simulink model "gm_uz_pmsm_model_6LUT_pd_vnl"  (R2023b)
settings: Solver=FixedStepAuto  StartTime=0.0  StopTime=0.05  RelTol=1e-3
PreLoadFcn:
  | uz_pmsm_model_init_parameter
PostLoadFcn:
  | % Import the data from Excel for a lookup table
  | FluxMapData = readtable('C:\Users\Philipp\ultrazohm\ultrazohm_sw\ip_cores\uz_pmsm_model\FluxMapData_2023-05-26_13-07-57.csv');
  | % Row indices for lookup table
  | d_current_in_d_axis = FluxMapData(8:27,1:end);
  | % Column indices for lookup table
  | q_current_in_d_axis = FluxMapData(29:48,1:end);
  | % Output values for lookup table
  | d_Flux_d_axis = FluxMapData(50:69,1:end);
undefined symbols (not defined in the file or in its folder): ad1, ad2, ad3, ad4, ad5, ad6, aq1, aq2, aq3, aq4, aq5, aq6, d_current_d_Flux, d_current_q_Flux, entkopplung_dynamic, entkopplung_linear, entkopplung_static, Fid1_Giq1, Fid2_Giq2, Flux_d, Flux_q, friction_coefficient, inertia, Ki_Bo_d, Ki_Bo_q, Kp_Bo_d, Kp_Bo_q, L_d, L_q, Ldq, parameter_nachfuerung, polepair, praediktion_entkopplung_nonlinear, psi_pm, q_current_d_Flux, q_current_q_Flux, R_1, simulate_mechanical, simulate_nonlinear_modell, simulate_open_loop, static_friction_torque, tau_sum, ts, ts_regler
libraries: hdlmdlgenlib x21, simulink x2, slpidlib x2
(part 2 of 4)

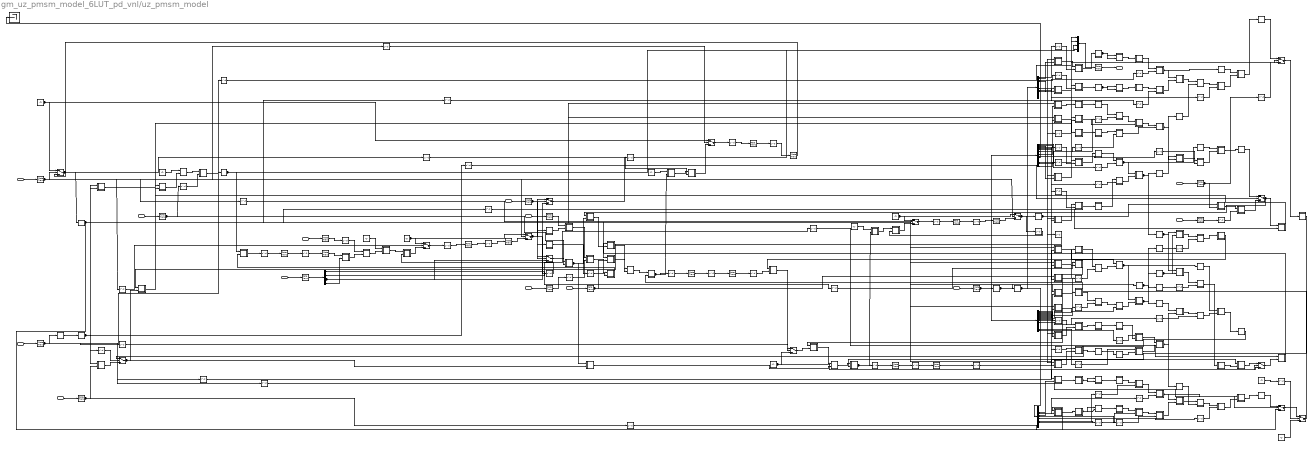
== system gm_uz_pmsm_model_6LUT_pd_vnl/uz_pmsm_model ==
  reset_integrators : Inport  OutDataTypeStr=boolean  PortDimensions=1  SampleTime=2e-06
  simulate_mechanical : Inport  Port=2  OutDataTypeStr=boolean  PortDimensions=1  SampleTime=2e-06
  simulate_nonlinear : Inport  Port=3  OutDataTypeStr=boolean  PortDimensions=1  SampleTime=2e-06
  reciprocal_J : Inport  Port=4  OutDataTypeStr=single  PortDimensions=1  SampleTime=2e-06
  mu : Inport  Port=5  OutDataTypeStr=single  PortDimensions=1  SampleTime=2e-06
  M_n0 : Inport  Port=6  OutDataTypeStr=single  PortDimensions=1  SampleTime=2e-06
  R1 : Inport  Port=7  OutDataTypeStr=single  PortDimensions=1  SampleTime=2e-06
  polepairs : Inport  Port=8  OutDataTypeStr=single  PortDimensions=1  SampleTime=2e-06
  Ld : Inport  Port=9  OutDataTypeStr=single  PortDimensions=1  SampleTime=2e-06
  Lq : Inport  Port=10  OutDataTypeStr=single  PortDimensions=1  SampleTime=2e-06
  psi_pm : Inport  Port=11  OutDataTypeStr=single  PortDimensions=1  SampleTime=2e-06
  fitting_parameters : Inport  Port=12  OutDataTypeStr=single  PortDimensions=[23]  SampleTime=2e-06
  inputs : Inport  Port=13  OutDataTypeStr=single  PortDimensions=[4]  SampleTime=2e-06
  Abs : Subsystem
      mask Display: disp('NFP\nabs');
  Constant : Constant  Value=single(0)  OutDataTypeStr=single  SampleTime=1e-08
  Delay : RateTransition  OutPortSampleTimeOpt=Multiple of input port sample time  OutPortSampleTimeMultiple=200
  Delay1_lowered : RateTransition  OutPortSampleTimeOpt=Multiple of input port sample time  OutPortSampleTimeMultiple=200
  Delay1_lowered1 : RateTransition  OutPortSampleTimeOpt=Multiple of input port sample time  OutPortSampleTimeMultiple=200
  Delay1_lowered2 : RateTransition  OutPortSampleTimeOpt=Multiple of input port sample time  OutPortSampleTimeMultiple=200
  Delay1_lowered_absorbed : Delay  DelayLength=0
  Delay1_lowered_absorbed1 : Delay  DelayLength=0
  Delay1_lowered_absorbed2 : Delay  DelayLength=0
  Delay_absorbed : Delay  DelayLength=0
  Divide : Subsystem
      mask Display: disp('NFP\nmul');
  Divide1 : Subsystem
      mask Display: disp('NFP\nmul');
  Divide_recip : Subsystem
      mask Display: disp('NFP\nmath');
  Factor : Subsystem
      mask Display: disp('NFP\nmul');
  Factor_const : Constant  Value=single(1.5)  OutDataTypeStr=single  SampleTime=1e-08
  From1 : hdlmdlgenlib/Buffer
  From2 : hdlmdlgenlib/Buffer
  From3 : hdlmdlgenlib/Buffer
  Gain : Subsystem
      mask Display: disp('NFP\nmul');
  Gain7 : Subsystem
      mask Display: disp('NFP\nmul');
  Gain71 : Subsystem
      mask Display: disp('NFP\nmul');
  Gain7_const : Constant  Value=single(2e-06)  OutDataTypeStr=single  SampleTime=1e-08
  Gain7_const1 : Constant  Value=single(2e-06)  OutDataTypeStr=single  SampleTime=1e-08
  Gain_const : Constant  Value=single(2e-06)  OutDataTypeStr=single  SampleTime=1e-08
  Gain_unaryminus : Subsystem
      mask Display: disp('NFP\numinus');
  Gain_unaryminus1 : Subsystem
      mask Display: disp('NFP\numinus');
  Goto1 : hdlmdlgenlib/Buffer
  Goto2 : hdlmdlgenlib/Buffer
  Initial_Val : Constant  Value=single(0)  OutDataTypeStr=single  SampleTime=1e-08
  Initial_Val1 : Constant  Value=single(0)  OutDataTypeStr=single  SampleTime=1e-08
  Initial_Val2 : Constant  Value=single(0)  OutDataTypeStr=single  SampleTime=1e-08
  Ldd : hdlmdlgenlib/Buffer
  Log : Subsystem
      mask Display: disp('NFP\nmath');
  Log1 : Subsystem
      mask Display: disp('NFP\nmath');
  Log11 : Subsystem
      mask Display: disp('NFP\nmath');
  Log2 : Subsystem
      mask Display: disp('NFP\nmath');
  Lqq : hdlmdlgenlib/Buffer
  Product : Subsystem
      mask Display: disp('NFP\nmul');
  Product1 : Subsystem
      mask Display: disp('NFP\nmul');
  Product10 : Subsystem
      mask Display: disp('NFP\nmul');
  Product101 : Subsystem
      mask Display: disp('NFP\nmul');
  Product102 : Subsystem
      mask Display: disp('NFP\nmul');
  Product103 : Subsystem
      mask Display: disp('NFP\nmul');
  Product104 : Subsystem
      mask Display: disp('NFP\nmul');
  Product11 : Subsystem
      mask Display: disp('NFP\nmul');
  Product110 : Subsystem
      mask Display: disp('NFP\nmul');
  Product111 : Subsystem
      mask Display: disp('NFP\nmul');
  Product12 : Subsystem
      mask Display: disp('NFP\nmul');
  Product121 : Subsystem
      mask Display: disp('NFP\nmul');
  Product122 : Subsystem
      mask Display: disp('NFP\nmul');
  Product13 : Subsystem
      mask Display: disp('NFP\nmul');
  Product131 : Subsystem
      mask Display: disp('NFP\nmul');
  Product14 : Subsystem
      mask Display: disp('NFP\nmul');
  Product141 : Subsystem
      mask Display: disp('NFP\nmul');
  Product142 : Subsystem
      mask Display: disp('NFP\nmul');
  Product15 : Subsystem
      mask Display: disp('NFP\nmul');
  Product151 : Subsystem
      mask Display: disp('NFP\nmul');
  Product16 : Subsystem
      mask Display: disp('NFP\nmul');
  Product17 : Subsystem
      mask Display: disp('NFP\nmul');
  Product18 : Subsystem
      mask Display: disp('NFP\nmul');
  Product19 : Subsystem
      mask Display: disp('NFP\nmul');
  Product2 : Subsystem
      mask Display: disp('NFP\nmul');
  Product20 : Subsystem
      mask Display: disp('NFP\nmul');
  Product201 : Subsystem
      mask Display: disp('NFP\nmul');
  Product202 : Subsystem
      mask Display: disp('NFP\nmul');
  Product203 : Subsystem
      mask Display: disp('NFP\nmul');
  Product204 : Subsystem
      mask Display: disp('NFP\nmul');
  Product205 : Subsystem
      mask Display: disp('NFP\nmul');
  Product206 : Subsystem
      mask Display: disp('NFP\nmul');
  Product207 : Subsystem
      mask Display: disp('NFP\nmul');
  Product21 : Subsystem
      mask Display: disp('NFP\nmul');
  Product22 : Subsystem
      mask Display: disp('NFP\nmul');
  Product23 : Subsystem
      mask Display: disp('NFP\nmul');
  Product24 : Subsystem
      mask Display: disp('NFP\nmul');
  Product25 : Subsystem
      mask Display: disp('NFP\nmul');
  Product3 : Subsystem
      mask Display: disp('NFP\nmul');
  Product31 : Subsystem
      mask Display: disp('NFP\nmul');
  Product32 : Subsystem
      mask Display: disp('NFP\nmul');
  Product33 : Subsystem
      mask Display: disp('NFP\nmul');
  Product34 : Subsystem
      mask Display: disp('NFP\nmul');
  Product35 : Subsystem
      mask Display: disp('NFP\nmul');
  Product4 : Subsystem
      mask Display: disp('NFP\nmul');
  Product41 : Subsystem
      mask Display: disp('NFP\nmul');
  Product42 : Subsystem
      mask Display: disp('NFP\nmul');
  Product43 : Subsystem
      mask Display: disp('NFP\nmul');
  Product5 : Subsystem
      mask Display: disp('NFP\nmul');
  Product51 : Subsystem
      mask Display: disp('NFP\nmul');
  Product52 : Subsystem
      mask Display: disp('NFP\nmul');
  Product6 : Subsystem
      mask Display: disp('NFP\nmul');
  Product61 : Subsystem
      mask Display: disp('NFP\nmul');
  Product7 : Subsystem
      mask Display: disp('NFP\nmul');
  Product71 : Subsystem
      mask Display: disp('NFP\nmul');
  Product8 : Subsystem
      mask Display: disp('NFP\nmul');
  Product9 : Subsystem
      mask Display: disp('NFP\nmul');
  Product91 : Subsystem
      mask Display: disp('NFP\nmul');
  Product92 : Subsystem
      mask Display: disp('NFP\nmul');
  Reciprocal1_recip : Subsystem
      mask Display: disp('NFP\nmath');
  Reciprocal1_recip1 : Subsystem
      mask Display: disp('NFP\nmath');
  Reciprocal_recip : Subsystem
      mask Display: disp('NFP\nmath');
  Reciprocal_recip1 : Subsystem
      mask Display: disp('NFP\nmath');
  Selector : Selector  IndexOptions=Index vector (dialog)  Indices=double(13)  OutputSizes=double(1)
  Selector1 : Selector  IndexOptions=Index vector (dialog)  Indices=double(14)  OutputSizes=double(1)
  Sign1 : Subsystem
      mask Display: disp('NFP\nsignum');
  Sum : Subsystem
      mask Display: disp('NFP\nadd');
  Sum1 : Subsystem
      mask Display: disp('NFP\nadd');
  Sum10 : Subsystem
      mask Display: disp('NFP\nadd');
  Sum101 : Subsystem
      mask Display: disp('NFP\nadd');
  Sum11 : Subsystem
      mask Display: disp('NFP\nadd');
  Sum12 : Subsystem
      mask Display: disp('NFP\nadd');
  Sum13 : Subsystem
      mask Display: disp('NFP\nadd');
  Sum14 : Subsystem
      mask Display: disp('NFP\nadd');
  Sum2 : Subsystem
      mask Display: disp('NFP\nadd');
  Sum21 : Subsystem
      mask Display: disp('NFP\nadd');
  Sum22 : Subsystem
      mask Display: disp('NFP\nadd');
  Sum23 : Subsystem
      mask Display: disp('NFP\nadd');
  Sum3 : Subsystem
      mask Display: disp('NFP\nadd');
  Sum31 : Subsystem
      mask Display: disp('NFP\nadd');
  Sum32 : Subsystem
      mask Display: disp('NFP\nadd');
  Sum33 : Subsystem
      mask Display: disp('NFP\nadd');
  Sum3_stage2 : Subsystem
      mask Display: disp('NFP\nadd');
  Sum3_stage21 : Subsystem
      mask Display: disp('NFP\nadd');
  Sum3_stage3 : Subsystem
      mask Display: disp('NFP\nadd');
  Sum3_stage31 : Subsystem
      mask Display: disp('NFP\nadd');
  Sum3_stage4 : Subsystem
      mask Display: disp('NFP\nadd');
  Sum4 : Subsystem
      mask Display: disp('NFP\nadd');
  Sum41 : Subsystem
      mask Display: disp('NFP\nadd');
  Sum42 : Subsystem
      mask Display: disp('NFP\nadd');
  Sum4_stage2 : Subsystem
      mask Display: disp('NFP\nadd');
  Sum4_stage3 : Subsystem
      mask Display: disp('NFP\nadd');
  Sum4_stage4 : Subsystem
      mask Display: disp('NFP\nadd');
  Sum5 : Subsystem
      mask Display: disp('NFP\nadd');
  Sum51 : Subsystem
      mask Display: disp('NFP\nadd');
  Sum52 : Subsystem
      mask Display: disp('NFP\nadd');
  Sum53 : Subsystem
      mask Display: disp('NFP\nadd');
  Sum6 : Subsystem
      mask Display: disp('NFP\nadd');
  Sum7 : Subsystem
      mask Display: disp('NFP\nadd');
  Sum71 : Subsystem
      mask Display: disp('NFP\nadd');
  Sum8 : Subsystem
      mask Display: disp('NFP\nadd');
  Switch{,1..6,11} (8 alike) : Switch  Criteria=u2 ~= 0  Threshold=double(0)  OutDataTypeStr=single  SampleTime=1e-08  SaturateOnIntegerOverflow=off  InputSameDT=off
  Tanh : Subsystem
      mask Display: disp('NFP\ntrig');
  Tanh1 : Subsystem
      mask Display: disp('NFP\ntrig');
  Tanh11 : Subsystem
      mask Display: disp('NFP\ntrig');
  Tanh12 : Subsystem
      mask Display: disp('NFP\ntrig');
  Tanh13 : Subsystem
      mask Display: disp('NFP\ntrig');
  Tanh2 : Subsystem
      mask Display: disp('NFP\ntrig');
  Tanh21 : Subsystem
      mask Display: disp('NFP\ntrig');
  Tanh3 : Subsystem
      mask Display: disp('NFP\ntrig');
  Tanh31 : Subsystem
      mask Display: disp('NFP\ntrig');
  Tanh4 : Subsystem
      mask Display: disp('NFP\ntrig');
  Tanh41 : Subsystem
      mask Display: disp('NFP\ntrig');
  Tanh5 : Subsystem
      mask Display: disp('NFP\ntrig');
  Unit Delay : RateTransition  OutPortSampleTimeOpt=Multiple of input port sample time  OutPortSampleTimeMultiple=200
  Unit Delay1 : RateTransition  OutPortSampleTimeOpt=Multiple of input port sample time  OutPortSampleTimeMultiple=200
  Unit Delay1_absorbed : Delay  DelayLength=0
  Unit Delay_absorbed : Delay  DelayLength=0
  crp_out_delay{,1..5} (6 alike) : Delay  DelayLength=double(1)  InitialCondition=0  SampleTime=1e-08
  default_value : Constant  Value=double(1)  OutDataTypeStr=single  SampleTime=1e-08
  delayMatch{,1..49,51..55} (55 alike) : Delay  DelayLength=double(1)  InitialCondition=0  SampleTime=1e-08
  delayMatch50 : Delay  DelayLength=double(97)  InitialCondition=0  SampleTime=1e-08
  fitting_parameters_13_term13 : Terminator
  i_q : hdlmdlgenlib/Buffer
  in0_repeat : RateTransition  Integrity=off  Deterministic=off  OutPortSampleTimeOpt=Multiple of input port sample time  OutPortSampleTimeMultiple=1/200
  in10_repeat : RateTransition  Integrity=off  Deterministic=off  OutPortSampleTimeOpt=Multiple of input port sample time  OutPortSampleTimeMultiple=1/200
  in11_repeat : RateTransition  Integrity=off  Deterministic=off  OutPortSampleTimeOpt=Multiple of input port sample time  OutPortSampleTimeMultiple=1/200
  in12_repeat : RateTransition  Integrity=off  Deterministic=off  OutPortSampleTimeOpt=Multiple of input port sample time  OutPortSampleTimeMultiple=1/200
  in13_repeat : RateTransition  Integrity=off  Deterministic=off  OutPortSampleTimeOpt=Multiple of input port sample time  OutPortSampleTimeMultiple=1/200
  in14_repeat : RateTransition  Integrity=off  Deterministic=off  OutPortSampleTimeOpt=Multiple of input port sample time  OutPortSampleTimeMultiple=1/200
  in15_repeat : RateTransition  Integrity=off  Deterministic=off  OutPortSampleTimeOpt=Multiple of input port sample time  OutPortSampleTimeMultiple=1/200
  in16_repeat : RateTransition  Integrity=off  Deterministic=off  OutPortSampleTimeOpt=Multiple of input port sample time  OutPortSampleTimeMultiple=1/200
  in17_repeat : RateTransition  Integrity=off  Deterministic=off  OutPortSampleTimeOpt=Multiple of input port sample time  OutPortSampleTimeMultiple=1/200
  in18_repeat : RateTransition  Integrity=off  Deterministic=off  OutPortSampleTimeOpt=Multiple of input port sample time  OutPortSampleTimeMultiple=1/200
  in1_repeat : RateTransition  Integrity=off  Deterministic=off  OutPortSampleTimeOpt=Multiple of input port sample time  OutPortSampleTimeMultiple=1/200
  in2_repeat : RateTransition  Integrity=off  Deterministic=off  OutPortSampleTimeOpt=Multiple of input port sample time  OutPortSampleTimeMultiple=1/200
  in3_repeat : RateTransition  Integrity=off  Deterministic=off  OutPortSampleTimeOpt=Multiple of input port sample time  OutPortSampleTimeMultiple=1/200
  in4_repeat : RateTransition  Integrity=off  Deterministic=off  OutPortSampleTimeOpt=Multiple of input port sample time  OutPortSampleTimeMultiple=1/200
  in5_repeat : RateTransition  Integrity=off  Deterministic=off  OutPortSampleTimeOpt=Multiple of input port sample time  OutPortSampleTimeMultiple=1/200
  in6_repeat : RateTransition  Integrity=off  Deterministic=off  OutPortSampleTimeOpt=Multiple of input port sample time  OutPortSampleTimeMultiple=1/200
  in7_repeat : RateTransition  Integrity=off  Deterministic=off  OutPortSampleTimeOpt=Multiple of input port sample time  OutPortSampleTimeMultiple=1/200
  in8_repeat : RateTransition  Integrity=off  Deterministic=off  OutPortSampleTimeOpt=Multiple of input port sample time  OutPortSampleTimeMultiple=1/200
  in9_repeat : RateTransition  Integrity=off  Deterministic=off  OutPortSampleTimeOpt=Multiple of input port sample time  OutPortSampleTimeMultiple=1/200
  mux : Mux
  psi_d_approx : hdlmdlgenlib/Buffer
  psi_q_approx : hdlmdlgenlib/Buffer
  reset_in : Switch  Criteria=u2 ~= 0  Threshold=double(0)  OutDataTypeStr=single  SampleTime=1e-08  SaturateOnIntegerOverflow=off  InputSameDT=off
  reset_in1 : Switch  Criteria=u2 ~= 0  Threshold=double(0)  OutDataTypeStr=single  SampleTime=1e-08  SaturateOnIntegerOverflow=off  InputSameDT=off
  reset_in2 : Switch  Criteria=u2 ~= 0  Threshold=double(0)  OutDataTypeStr=single  SampleTime=1e-08  SaturateOnIntegerOverflow=off  InputSameDT=off
  reset_out : Switch  Criteria=u2 ~= 0  Threshold=double(0)  OutDataTypeStr=single  SampleTime=1e-08  SaturateOnIntegerOverflow=off  InputSameDT=off
  reset_out1 : Switch  Criteria=u2 ~= 0  Threshold=double(0)  OutDataTypeStr=single  SampleTime=1e-08  SaturateOnIntegerOverflow=off  InputSameDT=off
  reset_out2 : Switch  Criteria=u2 ~= 0  Threshold=double(0)  OutDataTypeStr=single  SampleTime=1e-08  SaturateOnIntegerOverflow=off  InputSameDT=off
  select_signal : Constant  Value=double(1)  OutDataTypeStr=boolean  SampleTime=1e-08
  t : RateTransition  OutPortSampleTimeOpt=Multiple of input port sample time  OutPortSampleTimeMultiple=200
  t{1..4} (4 alike) : Demux  Outputs=23
  t{6..16} (11 alike) : hdlmdlgenlib/Buffer
  t5 : Demux
  zero_protection : Switch  Criteria=u2 ~= 0  Threshold=double(0)  OutDataTypeStr=single  SampleTime=1e-08  SaturateOnIntegerOverflow=off  InputSameDT=off
  outputs : Outport  SampleTime=2e-06
  wires:
  default_value/1 -> zero_protection/3
  zero_protection/1 -> Divide1/2(In2)
  reset_out1/1 -> Switch/1, Switch11/1, Sign1/1(In1), Abs/1(In1), delayMatch54/1
  delayMatch55/1 -> reset_in1/2
  reset_out/1 -> delayMatch51/1, t9/1
  select_signal/1 -> delayMatch50/1
  Switch1/1 -> zero_protection/1
  delayMatch48/1 -> Switch1/2
  Selector1/1 -> delayMatch39/1
  Switch11/1 -> delayMatch36/1
  delayMatch34/1 -> mux/1
  delayMatch35/1 -> mux/2
  From3/1 -> delayMatch14/1, delayMatch30/1
  delayMatch52/1 -> reset_in/2
  reset_out2/1 -> delayMatch26/1, t11/1
  delayMatch41/1 -> Switch4/2
  delayMatch24/1 -> Switch2/2
  delayMatch30/1 -> Switch5/2
  Selector/1 -> delayMatch7/1
  delayMatch50/1 -> zero_protection/2
  Gain/1(Out1) -> Sum32/1(In1)
  Sum3_stage4/1(Out1) -> Divide/1(In1)
  Sum3_stage31/1(Out1) -> Sum3_stage4/1(In1)
  Sum3_stage21/1(Out1) -> Sum3_stage31/1(In1)
  Divide_recip/1(Out1) -> Divide/2(In2)
  Sum53/1(Out1) -> reset_in2/3
  Product43/1(Out1) -> Sum3_stage21/2(In2)
  Product35/1(Out1) -> Sum33/1(In1)
  Sum33/1(Out1) -> Factor/2(In2)
  Sum8/1(Out1) -> crp_out_delay2/1
  Product42/1(Out1) -> Sum8/2(In2)
  Sum52/1(Out1) -> Product42/1(In1)
  Product122/1(Out1) -> Sum52/1(In1)
  Abs/1(Out1) -> Product122/2(In2)
  Sum32/1(Out1) -> reset_in1/3
  Product111/1(Out1) -> Gain/2(In2)
  Sum14/1(Out1) -> Product111/2(In2)
  Sign1/1(Out1) -> delayMatch38/1
  Product131/1(Out1) -> Product34/1(In1), Product22/2(In2)
  Sum42/1(Out1) -> Sum23/1(In1), t16/1
  Sum23/1(Out1) -> t10/1, t15/1
  Product206/1(Out1) -> Product207/1(In1)
  Product121/1(Out1) -> Switch3/1
  Sum4_stage4/1(Out1) -> Divide1/1(In1)
  Sum4_stage3/1(Out1) -> Sum4_stage4/1(In1)
  Sum4_stage2/1(Out1) -> Sum4_stage3/1(In1)
  Sum51/1(Out1) -> reset_in/3
  Product25/1(Out1) -> Tanh13/1(In1)
  Tanh13/1(Out1) -> Product151/1(In1), Product151/2(In2)
  Product151/1(Out1) -> Reciprocal1_recip1/1(In1)
  Reciprocal1_recip1/1(Out1) -> Product33/1(In1)
  Sum41/1(Out1) -> Sum22/2(In2)
  Sum22/1(Out1) -> Product204/1(In1)
  Product204/1(Out1) -> Product205/1(In1)
  Product202/1(Out1) -> Product203/1(In1)
  Tanh12/1(Out1) -> Product32/1(In1)
  Product24/1(Out1) -> Tanh12/1(In1)
  Sum13/1(Out1) -> Sum23/2(In2)
  Product61/1(Out1) -> Sum13/2(In2)
  Product52/1(Out1) -> Sum42/1(In1)
  Product110/1(Out1) -> Sum42/2(In2)
  Tanh5/1(Out1) -> Product110/1(In1)
  Product19/1(Out1) -> Tanh5/1(In1)
  Tanh21/1(Out1) -> Log11/1(In1)
  Log11/1(Out1) -> Product91/2(In2)
  Product91/1(Out1) -> Sum5/2(In2)
  Tanh41/1(Out1) -> Log2/1(In1)
  Log2/1(Out1) -> Product41/2(In2)
  Product41/1(Out1) -> Sum5/1(In1)
  Sum12/1(Out1) -> Sum10/1(In1), Sum22/1(In1)
  Reciprocal_recip1/1(Out1) -> Product18/1(In1)
  Product142/1(Out1) -> Reciprocal_recip1/1(In1)
  Tanh31/1(Out1) -> Product142/1(In1), Product142/2(In2)
  Product17/1(Out1) -> Tanh31/1(In1)
  Product16/1(Out1) -> Tanh4/1(In1)
  Sum4/1(Out1) -> Product16/1(In1)
  Tanh4/1(Out1) -> Product141/1(In1), Product141/2(In2)
  Product141/1(Out1) -> Reciprocal_recip/1(In1)
  Reciprocal_recip/1(Out1) -> Product14/1(In1)
  Product14/1(Out1) -> Sum2/1(In1), t12/1
  Product102/1(Out1) -> Product103/1(In1)
  Sum3_stage2/1(Out1) -> Sum3_stage3/1(In1)
  Product10/1(Out1) -> Product101/1(In1)
  Product13/1(Out1) -> Sum21/1(In1), t14/1
  Sum21/1(Out1) -> t8/1, t13/1
  Tanh11/1(Out1) -> Product31/1(In1)
  Product23/1(Out1) -> Tanh11/1(In1)
  Sum11/1(Out1) -> Product23/1(In1)
  Product7/1(Out1) -> Sum3_stage2/2(In2)
  Product8/1(Out1) -> Product7/1(In1)
  Product51/1(Out1) -> Tanh3/1(In1)
  Tanh3/1(Out1) -> Log1/1(In1)
  Log1/1(Out1) -> Product12/1(In1)
  Product12/1(Out1) -> Sum3_stage3/2(In2)
  Product4/1(Out1) -> Tanh2/1(In1)
  Tanh2/1(Out1) -> Log/1(In1)
  Log/1(Out1) -> Product6/1(In1)
  Product6/1(Out1) -> Sum3_stage2/1(In1)
  Product/1(Out1) -> Tanh/1(In1)
  Sum3/1(Out1) -> Product/1(In1)
  Tanh/1(Out1) -> Product13/1(In1)
  Product201/1(Out1) -> Gain_unaryminus/1(In1)
  Product20/1(Out1) -> Product201/1(In1)
  Product11/1(Out1) -> Switch4/1
  Sum/1(Out1) -> Switch5/3
  Product5/1(Out1) -> Sum/1(In1)
  Reciprocal1_recip/1(Out1) -> Product3/1(In1)
  Product15/1(Out1) -> Reciprocal1_recip/1(In1)
  Tanh1/1(Out1) -> Product15/1(In1), Product15/2(In2)
  Product21/1(Out1) -> Tanh1/1(In1)
  Sum1/1(Out1) -> Product21/1(In1)
  Product9/1(Out1) -> Sum4_stage4/2(In2)
  Product1/1(Out1) -> Switch6/3
  Product2/1(Out1) -> Sum33/2(In2)
  Gain7_const1/1 -> Gain71/1(In1)
  Factor_const/1 -> Factor/1(In1)
  Gain_const/1 -> Gain/1(In1)
  Gain7_const/1 -> Gain7/1(In1)
  t5/2 -> delayMatch42/1
  t5/1 -> delayMatch/1
  t4/22 -> delayMatch10/1
  t4/21 -> delayMatch12/1
  t4/14 -> delayMatch13/1
  t4/10 -> delayMatch6/1
  t4/7 -> delayMatch5/1
  t4/5 -> delayMatch11/1
  t4/2 -> delayMatch9/1
  t3/18 -> delayMatch43/1
  t3/17 -> delayMatch45/1
  t3/14 -> delayMatch47/1
  t3/12 -> delayMatch46/1
  t3/9 -> delayMatch44/1
  t2/16 -> delayMatch16/1
  t2/15 -> delayMatch18/1
  t2/13 -> delayMatch22/1
  t2/5 -> delayMatch17/1
  t2/2 -> delayMatch15/1
  t1/23 -> delayMatch20/1
  t1/20 -> delayMatch19/1
  t1/19 -> delayMatch21/1
  t1/14 -> fitting_parameters_13_term13/1
  t1/13 -> delayMatch28/1
  t1/5 -> delayMatch3/1
  t1/4 -> delayMatch4/1
  t1/2 -> delayMatch1/1
  t1/1 -> delayMatch2/1
  delayMatch37/1 -> Sum52/2(In2)
  delayMatch53/1 -> Product111/1(In1)
  delayMatch33/1 -> Product92/2(In2)
  delayMatch8/1 -> Product121/2(In2)
  delayMatch27/1 -> reset_in2/2
  delayMatch40/1 -> Product11/1(In1)
  delayMatch29/1 -> Sum/2(In2)
  delayMatch25/1 -> Switch2/3
  delayMatch49/1 -> Switch1/3
  delayMatch23/1 -> Switch3/2
  t5/4 -> Sum14/2(In2)
  t5/3 -> Switch/3, Switch11/3
  delayMatch42/1 -> Sum4_stage2/1(In1)
  delayMatch/1 -> Sum3_stage21/1(In1)
  Divide/1(Out1) -> crp_out_delay/1, Gain71/2(In2)
  Gain71/1(Out1) -> Sum53/1(In1)
  reset_in2/1 -> crp_out_delay1/1
  Initial_Val2/1 -> reset_in2/1, reset_out2/1
  delayMatch26/1 -> Sum53/2(In2)
  t11/1 -> delayMatch32/1, delayMatch34/1, Sum1/1(In1), Product5/1(In1), Sum3/1(In1), Sum11/1(In1), Sum4/1(In1), Sum31/1(In1), Sum6/1(In1), Product43/2(In2)
  delayMatch32/1 -> Product2/1(In1)
  delayMatch31/1 -> Product35/2(In2)
  Factor/1(Out1) -> Product92/1(In1)
  Product92/1(Out1) -> i_q/1
  i_q/1 -> mux/3, Sum8/1(In1)
  delayMatch54/1 -> Sum32/2(In2)
  reset_in1/1 -> crp_out_delay5/1
  Initial_Val1/1 -> reset_in1/1, reset_out1/1
  delayMatch38/1 -> Product42/2(In2)
  delayMatch36/1 -> mux/4
  Switch/1 -> Product131/1(In1)
  Product34/1(Out1) -> Sum3_stage4/2(In2)
  Switch6/1 -> Product2/2(In2), Product34/2(In2)
  psi_q_approx/1 -> Switch6/1
  Sum101/1(Out1) -> psi_q_approx/1
  t16/1 -> Sum101/1(In1)
  t15/1 -> Product202/1(In1)
  t10/1 -> Product20/2(In2), Product206/2(In2)
  Product207/1(Out1) -> Gain_unaryminus1/1(In1)
  Gain_unaryminus1/1(Out1) -> Product121/1(In1)
  Switch3/1 -> Sum3_stage31/2(In2)
  Constant/1 -> Switch4/3, Switch3/3
  Switch4/1 -> Sum4_stage2/2(In2)
  Divide1/1(Out1) -> crp_out_delay3/1, Gain7/2(In2)
  Gain7/1(Out1) -> Sum51/1(In1)
  reset_in/1 -> crp_out_delay4/1
  Initial_Val/1 -> reset_in/1, reset_out/1
  delayMatch51/1 -> Sum51/2(In2)
  t9/1 -> delayMatch31/1, delayMatch35/1, Product1/1(In1), Product9/1(In1), Product4/1(In1), Product51/1(In1), Product8/1(In1), Product8/2(In2), Product17/1(In1), Product19/1(In1), Product52/1(In1), Product61/1(In1), Product24/1(In1), Product25/1(In1)
  Product33/1(Out1) -> Sum41/1(In1)
  Product205/1(Out1) -> Sum10/2(In2)
  t6/1 -> Product204/2(In2)
  Sum5/1(Out1) -> Product202/2(In2), t6/1
  Product203/1(Out1) -> Sum101/2(In2)
  delayMatch10/1 -> Product41/1(In1)
  delayMatch12/1 -> Product91/1(In1)
  delayMatch13/1 -> Product203/2(In2)
  t4/12 -> Product61/2(In2)
  t4/11 -> Product24/2(In2)
  delayMatch6/1 -> Product32/2(In2)
  t4/9 -> Product52/2(In2)
  t4/8 -> Product19/2(In2)
  delayMatch5/1 -> Product110/2(In2)
  t4/6 -> Sum6/2(In2)
  delayMatch11/1 -> Product104/1(In1)
  t4/3 -> Sum31/2(In2)
  delayMatch9/1 -> Product71/1(In1)
  Product32/1(Out1) -> Sum13/1(In1)
  Product104/1(Out1) -> Tanh21/1(In1)
  Sum6/1(Out1) -> Product104/2(In2)
  Product71/1(Out1) -> Tanh41/1(In1)
  Sum31/1(Out1) -> Product71/2(In2)
  Sum10/1(Out1) -> Lqq/1
  Product18/1(Out1) -> Sum12/1(In1)
  delayMatch43/1 -> Product18/2(In2)
  delayMatch45/1 -> Product33/2(In2)
  delayMatch47/1 -> Product205/2(In2)
  delayMatch46/1 -> Sum41/2(In2)
  t3/11 -> Product25/2(In2)
  delayMatch44/1 -> Sum12/2(In2)
  t3/8 -> Product17/2(In2)
  From1/1 -> t2/1, t3/1
  delayMatch16/1 -> Product14/2(In2)
  delayMatch18/1 -> Product3/2(In2)
  delayMatch22/1 -> Product103/2(In2)
  t2/6 -> Sum1/2(In2)
  delayMatch17/1 -> Product21/2(In2)
  t2/3 -> Sum4/2(In2)
  delayMatch15/1 -> Product16/2(In2)
  t12/1 -> Sum71/1(In1)
  Sum71/1(Out1) -> Ldd/1
  Product103/1(Out1) -> Sum71/2(In2)
  t7/1 -> Product102/2(In2)
  Sum3_stage3/1(Out1) -> Product10/2(In2), t7/1
  Product101/1(Out1) -> Sum7/2(In2)
  Sum7/1(Out1) -> psi_d_approx/1
  t14/1 -> Sum7/1(In1)
  t13/1 -> Product10/1(In1)
  Product31/1(Out1) -> Sum21/2(In2)
  delayMatch20/1 -> Product7/2(In2)
  delayMatch19/1 -> Product6/2(In2)
  delayMatch21/1 -> Product12/2(In2)
  delayMatch28/1 -> Product101/2(In2)
  t1/11 -> Product51/2(In2)
  t1/8 -> Product4/2(In2)
  t1/6 -> Sum11/2(In2)
  delayMatch3/1 -> Product23/2(In2)
  delayMatch4/1 -> Product31/2(In2)
  t1/3 -> Sum3/2(In2)
  delayMatch1/1 -> Product/2(In2)
  delayMatch2/1 -> Product13/2(In2)
  t8/1 -> Product20/1(In1), Product206/1(In1)
  delayMatch39/1 -> Product201/2(In2)
  From2/1 -> Selector/1, Selector1/1
  Goto1/1 -> From1/1, From2/1
  delayMatch7/1 -> Product207/2(In2)
  Gain_unaryminus/1(Out1) -> Product11/2(In2)
  psi_d_approx/1 -> Switch5/1
  Switch5/1 -> Product35/1(In1), Product22/1(In1)
  delayMatch14/1 -> Switch6/2
  Goto2/1 -> From3/1
  Product22/1(Out1) -> Sum4_stage3/2(In2)
  Sum2/1(Out1) -> Product102/1(In1)
  Product3/1(Out1) -> Sum2/2(In2)
  Ldd/1 -> Switch2/1
  Switch2/1 -> Divide_recip/1(In1)
  Lqq/1 -> Switch1/1
  crp_out_delay5/1 -> Delay1_lowered1/1
  crp_out_delay4/1 -> Delay1_lowered2/1
  crp_out_delay3/1 -> Unit Delay1/1
  crp_out_delay2/1 -> Delay/1
  crp_out_delay1/1 -> Delay1_lowered/1
  crp_out_delay/1 -> Unit Delay/1
  in6_repeat/1 -> delayMatch40/1
  Unit Delay_absorbed/1 -> in6_repeat/1
  Unit Delay/1 -> Unit Delay_absorbed/1
  in9_repeat/1 -> reset_out/3
  Delay1_lowered_absorbed2/1 -> in9_repeat/1
  Delay1_lowered2/1 -> Delay1_lowered_absorbed2/1
  in10_repeat/1 -> delayMatch8/1
  Unit Delay1_absorbed/1 -> in10_repeat/1
  Unit Delay1/1 -> Unit Delay1_absorbed/1
  in14_repeat/1 -> Sum14/1(In1)
  Delay_absorbed/1 -> in14_repeat/1
  Delay/1 -> Delay_absorbed/1
  in15_repeat/1 -> reset_out1/3
  Delay1_lowered_absorbed1/1 -> in15_repeat/1
  Delay1_lowered1/1 -> Delay1_lowered_absorbed1/1
  in17_repeat/1 -> reset_out2/3
  Delay1_lowered_absorbed/1 -> in17_repeat/1
  Delay1_lowered/1 -> Delay1_lowered_absorbed/1
  mux/1 -> t/1
  in18_repeat/1 -> t5/1
  in16_repeat/1 -> delayMatch37/1
  in13_repeat/1 -> delayMatch53/1
  in12_repeat/1 -> Switch/2, Switch11/2
  in11_repeat/1 -> Product131/2(In2), delayMatch33/1
  in8_repeat/1 -> reset_out/2, reset_out2/2, reset_out1/2, delayMatch27/1, delayMatch52/1, delayMatch55/1
  in7_repeat/1 -> Goto1/1, t1/1, t4/1
  in5_repeat/1 -> delayMatch29/1
  in4_repeat/1 -> Product5/2(In2), delayMatch25/1
  in3_repeat/1 -> Product9/2(In2), Product43/1(In1)
  in2_repeat/1 -> Product1/2(In2), delayMatch49/1
  in1_repeat/1 -> Goto2/1, delayMatch23/1, delayMatch24/1, delayMatch41/1, delayMatch48/1
  in0_repeat/1 -> Product122/1(In1)
  t/1 -> outputs/1
  inputs/1 -> in18_repeat/1
  fitting_parameters/1 -> in7_repeat/1
  psi_pm/1 -> in5_repeat/1
  Lq/1 -> in2_repeat/1
  Ld/1 -> in4_repeat/1
  polepairs/1 -> in11_repeat/1
  R1/1 -> in3_repeat/1
  M_n0/1 -> in16_repeat/1
  mu/1 -> in0_repeat/1
  reciprocal_J/1 -> in13_repeat/1
  simulate_nonlinear/1 -> in1_repeat/1
  simulate_mechanical/1 -> in12_repeat/1
  reset_integrators/1 -> in8_repeat/1

== system gm_uz_pmsm_model_6LUT_pd_vnl/uz_pmsm_model_vnl ==
  reset_integrators : Inport
  simulate_mechanical : Inport  Port=2
  simulate_nonlinear : Inport  Port=3
  reciprocal_J : Inport  Port=4
  mu : Inport  Port=5
  M_n0 : Inport  Port=6
  R1 : Inport  Port=7
  polepairs : Inport  Port=8
  Ld : Inport  Port=9
  Lq : Inport  Port=10
  psi_pm : Inport  Port=11
  fitting_parameters : Inport  Port=12
  inputs : Inport  Port=13
  Demux : Demux
  Mux : Mux
  Switch : Switch  Criteria=u2 ~= 0  SaturateOnIntegerOverflow=off  InputSameDT=off
  Switch1 : Switch  Criteria=u2 ~= 0  SaturateOnIntegerOverflow=off  InputSameDT=off
  mechanical_system : Subsystem
  pmsm : Subsystem
  torque_calculation : Subsystem
  outputs : Outport
  wires:
  fitting_parameters/1 -> pmsm/10(fitting_parameters)
  reciprocal_J/1 -> mechanical_system/5(reciprocal_J)
  M_n0/1 -> mechanical_system/4(M_n0)
  mu/1 -> mechanical_system/3(mu)
  psi_pm/1 -> pmsm/9(psi_pm)
  Lq/1 -> pmsm/8(Lq)
  Ld/1 -> pmsm/7(Ld)
  polepairs/1 -> pmsm/6(polepairs1), torque_calculation/4(polepairs)
  R1/1 -> pmsm/5(R2)
  simulate_nonlinear/1 -> pmsm/2(simulate_nonlinear)
  Mux/1 -> outputs/1
  inputs/1 -> Demux/1
  torque_calculation/1(M_Mi) -> Mux/3, mechanical_system/2(M_Mi)  "i_q"
  Switch1/1 -> Mux/4  "i_q"
  pmsm/1(I_d1) -> torque_calculation/1(I_d), Mux/1  "i_d"
  pmsm/4(I_q1) -> Mux/2, torque_calculation/5(I_q)  "i_q"
  mechanical_system/1(omega_mech) -> Switch1/1, Switch/1
  Demux/2 -> pmsm/4(u_q1)  "u_q"
  simulate_mechanical/1 -> Switch/2, Switch1/2
  Demux/1 -> pmsm/3(u_d1)  "u_d"
  pmsm/3(psi_q1) -> torque_calculation/3(psi_q)
  Demux/4 -> mechanical_system/6(load_torque)  "load_torque"
  pmsm/2(psi_d1) -> torque_calculation/2(psi_d)
  Switch/1 -> pmsm/11(omega_mech1)
  Demux/3 -> Switch/3, Switch1/3  "omega_mech"
  reset_integrators/1 -> mechanical_system/1(reset), pmsm/1(reset1)

== system gm_uz_pmsm_model_6LUT_pd_vnl/Compare/Assert_outputs ==
  cosim : Inport
  dut : Inport  Port=2
  AssertEq : Assertion  StopWhenAssertionFail=off
  Compare To Zero : simulink/Logic and Bit Operations/Compare To Zero  relop===  OutDataTypeStr=boolean
  Constant1 : Constant  Value=0  OutDataTypeStr=Inherit: Inherit via back propagation  SampleTime=-1
  Counter : simulink/Sources/Counter Free-Running  NumBits=32  tsamp=-1
  IgnoreCycles : Constant  Value=2  OutDataTypeStr=Inherit: Inherit via back propagation  SampleTime=-1
  RelErrCheck : Subsystem
  Relational Operator : RelationalOperator  Operator=<  OutDataTypeStr=boolean  InputSameDT=off
  Switch : Switch  Criteria=u2 ~= 0  SaturateOnIntegerOverflow=off  InputSameDT=off
  Switch1 : Switch  Criteria=u2 ~= 0  SaturateOnIntegerOverflow=off  InputSameDT=off
  compare: outputs : Scope  NumInputPorts=3
  wires:
  IgnoreCycles/1 -> Relational Operator/2
  Counter/1 -> Relational Operator/1
  dut/1 -> Switch/3  "dut ref"
  cosim/1 -> Switch1/3  "cosim"
  Relational Operator/1 -> Switch1/2, Switch/2
  Constant1/1 -> Switch1/1, Switch/1
  Switch/1 -> compare: outputs/2, RelErrCheck/2(In2)
  Switch1/1 -> compare: outputs/1, RelErrCheck/1(In1)
  RelErrCheck/1(Out1) -> AssertEq/1, Compare To Zero/1  "err"
  Compare To Zero/1 -> compare: outputs/3

== system gm_uz_pmsm_model_6LUT_pd_vnl/Compare/CleanupScopes ==

== system gm_uz_pmsm_model_6LUT_pd_vnl/Compare/Enable ==

== system gm_uz_pmsm_model_6LUT_pd_vnl/Current_Controller/Entkopplung_flags ==
  u_d_static : Inport
  u_q_static : Inport  Port=2
  u_d_praed : Inport  Port=3
  u_q_praed : Inport  Port=4
  u_d_lin : Inport  Port=5
  u_q_lin : Inport  Port=6
  u_d_dyn : Inport  Port=7
  u_q_dyn : Inport  Port=8
  0 : Constant  Value=0
  Switch{1..8} (8 alike) : Switch  Criteria=u2 > Threshold  SaturateOnIntegerOverflow=off  InputSameDT=off
  entkopplung_dynamic : Constant  Value=entkopplung_dynamic
  entkopplung_linear : Constant  Value=entkopplung_linear
  entkopplung_preadiktion : Constant  Value=praediktion_entkopplung_nonlinear
  entkopplung_static : Constant  Value=entkopplung_static
  u_d_entk : Outport
  u_q_entk : Outport  Port=2
  wires:
  Switch3/1 -> u_d_entk/1
  Switch4/1 -> Switch2/3
  entkopplung_preadiktion/1 -> Switch2/2, Switch3/2
  Switch1/1 -> Switch3/3
  u_d_praed/1 -> Switch3/1
  Switch2/1 -> u_q_entk/1
  u_q_praed/1 -> Switch2/1
  entkopplung_static/1 -> Switch4/2, Switch1/2
  u_d_static/1 -> Switch1/1
  u_d_lin/1 -> Switch5/1
  Switch5/1 -> Switch1/3
  entkopplung_linear/1 -> Switch6/2, Switch5/2
  entkopplung_dynamic/1 -> Switch8/2, Switch7/2
  0/1 -> Switch8/3, Switch7/3
  Switch6/1 -> Switch4/3
  u_q_static/1 -> Switch4/1
  u_q_lin/1 -> Switch6/1
  u_d_dyn/1 -> Switch7/1
  Switch8/1 -> Switch6/3
  u_q_dyn/1 -> Switch8/1
  Switch7/1 -> Switch5/3

== system gm_uz_pmsm_model_6LUT_pd_vnl/Current_Controller/Entkopplungen ==
  u_q : Inport
  u_d : Inport  Port=2
  uq : Inport  Port=3
  ud : Inport  Port=4
  i_d : Inport  Port=5
  psi_d_LUT : Inport  Port=6
  psi_q_LUT : Inport  Port=7
  Ldq_LUT : Inport  Port=8
  Lqd_LUT : Inport  Port=9
  i_q : Inport  Port=10
  omega_m : Inport  Port=11
  Lineare_Entkopplung : Subsystem
  decoupling_praediktion : Subsystem
  dynamic_nonlinear_entkopplung1 : Subsystem
  static_nonlinear_entkopplung : Subsystem
  u_d_static : Outport
  u_q_static : Outport  Port=2
  u_d_prae : Outport  Port=3
  u_q_prae : Outport  Port=4
  u_d_lin : Outport  Port=5
  u_q_lin : Outport  Port=6
  u_d_dyn : Outport  Port=7
  u_q_dyn1 : Outport  Port=8
  wires:
  psi_d_LUT/1 -> static_nonlinear_entkopplung/1(psi_d), dynamic_nonlinear_entkopplung1/3(psi_d), decoupling_praediktion/9(psi_d)
  omega_m/1 -> dynamic_nonlinear_entkopplung1/7(omega_m), Lineare_Entkopplung/3(omega_m), static_nonlinear_entkopplung/3(omega_m), decoupling_praediktion/5(omega_m)
  psi_q_LUT/1 -> dynamic_nonlinear_entkopplung1/4(psi_q), decoupling_praediktion/8(psi_q), static_nonlinear_entkopplung/2(psi_q)
  u_q/1 -> decoupling_praediktion/4(u_q_1)
  i_d/1 -> dynamic_nonlinear_entkopplung1/1(i_d), Lineare_Entkopplung/1(i_d), decoupling_praediktion/1(i_d)
  i_q/1 -> dynamic_nonlinear_entkopplung1/2(i_q), Lineare_Entkopplung/2(i_q), decoupling_praediktion/3(i_q)
  ud/1 -> decoupling_praediktion/6(u_d_k)
  uq/1 -> decoupling_praediktion/7(u_q_k)
  u_d/1 -> decoupling_praediktion/2(u_d_1)
  static_nonlinear_entkopplung/1(u_d) -> u_d_static/1
  Lineare_Entkopplung/1(u_d) -> u_d_lin/1
  static_nonlinear_entkopplung/2(u_q) -> u_q_static/1
  decoupling_praediktion/1(u_d_entk) -> u_d_prae/1
  Lineare_Entkopplung/2(u_q) -> u_q_lin/1
  decoupling_praediktion/2(u_q_entk) -> u_q_prae/1
  dynamic_nonlinear_entkopplung1/1(u_d) -> u_d_dyn/1
  dynamic_nonlinear_entkopplung1/2(u_q) -> u_q_dyn1/1
  Ldq_LUT/1 -> dynamic_nonlinear_entkopplung1/5(Ldq_LUT)
  Lqd_LUT/1 -> dynamic_nonlinear_entkopplung1/6(Lqd_LUT)

== system gm_uz_pmsm_model_6LUT_pd_vnl/Current_Controller/Psi_d_q ==
  I_d_set : Inport
  I_d : Inport  Port=2
  I_q_set : Inport  Port=3
  I_q : Inport  Port=4
  Flux_d Lookup Table : Lookup_n-D  BreakpointsForDimension1=d_current_d_Flux  BreakpointsForDimension2=q_current_d_Flux  BreakpointsForDimension3=[5, 7]  Table=Flux_d  InternalRulePriority=Speed  RndMeth=Simplest
      settings: InputPortMap=u0,u1
  Flux_d Lookup Table1 : Lookup_n-D  BreakpointsForDimension1=d_current_d_Flux  BreakpointsForDimension2=q_current_d_Flux  BreakpointsForDimension3=[5, 7]  Table=Flux_d  InternalRulePriority=Speed  RndMeth=Simplest
      settings: InputPortMap=u0,u1
  Flux_q Lookup Table1 : Lookup_n-D  BreakpointsForDimension1=d_current_q_Flux  BreakpointsForDimension2=q_current_q_Flux  BreakpointsForDimension3=[5, 7]  Table=Flux_q  InternalRulePriority=Speed  RndMeth=Simplest
      settings: InputPortMap=u0,u1
  Flux_q Lookup Table2 : Lookup_n-D  BreakpointsForDimension1=d_current_q_Flux  BreakpointsForDimension2=q_current_q_Flux  BreakpointsForDimension3=[5, 7]  Table=Flux_q  InternalRulePriority=Speed  RndMeth=Simplest
      settings: InputPortMap=u0,u1
  Ldq Lookup Table : Lookup_n-D  BreakpointsForDimension1=d_current_q_Flux  BreakpointsForDimension2=q_current_q_Flux  BreakpointsForDimension3=[5, 7]  Table=Ldq  ExtrapMethod=Clip  UseLastTableValue=on  InternalRulePriority=Speed  OutDataTypeStr=Inherit: Inherit from 'Table data'  RndMeth=Simplest
      settings: InputPortMap=u0,u1
  Lqd Lookup Table1 : Lookup_n-D  BreakpointsForDimension1=d_current_q_Flux  BreakpointsForDimension2=q_current_q_Flux  BreakpointsForDimension3=[5, 7]  Table=Ldq  ExtrapMethod=Clip  UseLastTableValue=on  InternalRulePriority=Speed  OutDataTypeStr=Inherit: Inherit from 'Table data'  RndMeth=Simplest
      settings: InputPortMap=u0,u1
  Scope : Scope  NumInputPorts=4
  psi_d_set : Outport
  psi_q_set : Outport  Port=2
  psi_d_LUT : Outport  Port=3
  psi_q_LUT : Outport  Port=4
  Ldq_LUT : Outport  Port=5
  Lqd_LUT : Outport  Port=6
  wires:
  I_d_set/1 -> Scope/1, Flux_d Lookup Table1/1
  I_q_set/1 -> Scope/2, Flux_q Lookup Table2/2
  Flux_d Lookup Table1/1 -> psi_d_set/1  "psi_d_set"
  Flux_q Lookup Table2/1 -> psi_q_set/1  "psi_q_set"
  Flux_d Lookup Table/1 -> psi_d_LUT/1  "psi_d_controller"
  Flux_q Lookup Table1/1 -> psi_q_LUT/1  "psi_q_controller"
  Ldq Lookup Table/1 -> Ldq_LUT/1  "Ldq_Karte"
  Lqd Lookup Table1/1 -> Lqd_LUT/1  "Ldq_Karte"
  I_d/1 -> Scope/3, Flux_q Lookup Table2/1, Lqd Lookup Table1/1, Ldq Lookup Table/1, Flux_q Lookup Table1/1, Flux_d Lookup Table/1
  I_q/1 -> Scope/4, Lqd Lookup Table1/2, Ldq Lookup Table/2, Flux_q Lookup Table1/2, Flux_d Lookup Table1/2, Flux_d Lookup Table/2

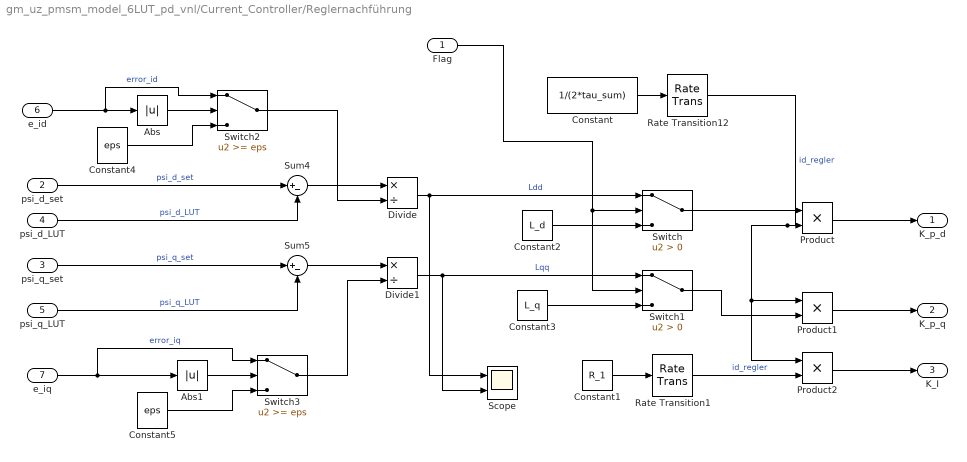
== system gm_uz_pmsm_model_6LUT_pd_vnl/Current_Controller/Reglernachführung ==
  Flag : Inport
  psi_d_set : Inport  Port=2
  psi_q_set : Inport  Port=3
  psi_d_LUT : Inport  Port=4
  psi_q_LUT : Inport  Port=5
  e_id : Inport  Port=6
  e_iq : Inport  Port=7
  Abs : Abs  SaturateOnIntegerOverflow=off
  Abs1 : Abs  SaturateOnIntegerOverflow=off
  Constant : Constant  Value=1/(2*tau_sum)
  Constant1 : Constant  Value=R_1
  Constant2 : Constant  Value=L_d
  Constant3 : Constant  Value=L_q
  Constant4 : Constant  Value=eps  SampleTime=ts_regler
  Constant5 : Constant  Value=eps  SampleTime=ts_regler
  Divide : Product  Inputs=*/
  Divide1 : Product  Inputs=*/
  Product : Product
  Product1 : Product
  Product2 : Product
  Rate Transition1 : RateTransition  OutPortSampleTime=ts_regler
  Rate Transition12 : RateTransition  OutPortSampleTime=ts_regler
  Scope : Scope  NumInputPorts=2
  Sum4 : Sum  Inputs=|+-
  Sum5 : Sum  Inputs=|+-
  Switch : Switch  Criteria=u2 > Threshold  SaturateOnIntegerOverflow=off  InputSameDT=off
  Switch1 : Switch  Criteria=u2 > Threshold  SaturateOnIntegerOverflow=off  InputSameDT=off
  Switch2 : Switch  Threshold=eps  SaturateOnIntegerOverflow=off  InputSameDT=off
  Switch3 : Switch  Threshold=eps  SaturateOnIntegerOverflow=off  InputSameDT=off
  K_p_d : Outport
  K_p_q : Outport  Port=2
  K_I : Outport  Port=3
  wires:
  Constant/1 -> Rate Transition12/1
  Product/1 -> K_p_d/1
  Product1/1 -> K_p_q/1
  Product2/1 -> K_I/1
  Constant1/1 -> Rate Transition1/1
  Rate Transition12/1 -> Product2/1, Product1/1, Product/2  "id_regler"
  Rate Transition1/1 -> Product2/2  "id_regler"
  Flag/1 -> Switch/2, Switch1/2
  Constant2/1 -> Switch/3
  Switch/1 -> Product/1
  Constant3/1 -> Switch1/3
  Switch1/1 -> Product1/2
  Sum4/1 -> Divide/1
  psi_q_LUT/1 -> Sum5/2  "psi_q_LUT"
  Sum5/1 -> Divide1/1
  psi_d_LUT/1 -> Sum4/2  "psi_d_LUT"
  psi_d_set/1 -> Sum4/1  "psi_d_set"
  psi_q_set/1 -> Sum5/1  "psi_q_set"
  Divide/1 -> Scope/1, Switch/1  "Ldd"
  Divide1/1 -> Scope/2, Switch1/1  "Lqq"
  e_id/1 -> Switch2/1, Abs/1  "error_id"
  Constant4/1 -> Switch2/3
  Abs/1 -> Switch2/2
  Switch2/1 -> Divide/2
  e_iq/1 -> Switch3/1, Abs1/1  "error_iq"
  Switch3/1 -> Divide1/2
  Abs1/1 -> Switch3/2
  Constant5/1 -> Switch3/3

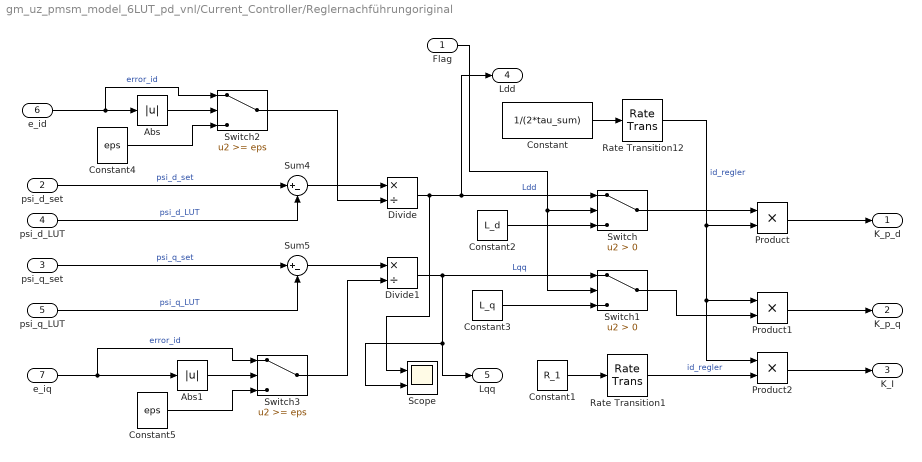
== system gm_uz_pmsm_model_6LUT_pd_vnl/Current_Controller/Reglernachführungoriginal ==
  Flag : Inport
  psi_d_set : Inport  Port=2
  psi_q_set : Inport  Port=3
  psi_d_LUT : Inport  Port=4
  psi_q_LUT : Inport  Port=5
  e_id : Inport  Port=6
  e_iq : Inport  Port=7
  Abs : Abs  SaturateOnIntegerOverflow=off
  Abs1 : Abs  SaturateOnIntegerOverflow=off
  Constant : Constant  Value=1/(2*tau_sum)
  Constant1 : Constant  Value=R_1
  Constant2 : Constant  Value=L_d
  Constant3 : Constant  Value=L_q
  Constant4 : Constant  Value=eps  SampleTime=ts_regler
  Constant5 : Constant  Value=eps  SampleTime=ts_regler
  Divide : Product  Inputs=*/
  Divide1 : Product  Inputs=*/
  Product : Product
  Product1 : Product
  Product2 : Product
  Rate Transition1 : RateTransition  OutPortSampleTime=ts_regler
  Rate Transition12 : RateTransition  OutPortSampleTime=ts_regler
  Scope : Scope  NumInputPorts=2
  Sum4 : Sum  Inputs=|+-
  Sum5 : Sum  Inputs=|+-
  Switch : Switch  Criteria=u2 > Threshold  SaturateOnIntegerOverflow=off  InputSameDT=off
  Switch1 : Switch  Criteria=u2 > Threshold  SaturateOnIntegerOverflow=off  InputSameDT=off
  Switch2 : Switch  Threshold=eps  SaturateOnIntegerOverflow=off  InputSameDT=off
  Switch3 : Switch  Threshold=eps  SaturateOnIntegerOverflow=off  InputSameDT=off
  K_p_d : Outport
  K_p_q : Outport  Port=2
  K_I : Outport  Port=3
  Ldd : Outport  Port=4
  Lqq : Outport  Port=5
  wires:
  Constant/1 -> Rate Transition12/1
  Product/1 -> K_p_d/1
  Product1/1 -> K_p_q/1
  Product2/1 -> K_I/1
  Constant1/1 -> Rate Transition1/1
  Rate Transition12/1 -> Product2/1, Product1/1, Product/2  "id_regler"
  Rate Transition1/1 -> Product2/2  "id_regler"
  Flag/1 -> Switch/2, Switch1/2
  Constant2/1 -> Switch/3
  Switch/1 -> Product/1
  Constant3/1 -> Switch1/3
  Switch1/1 -> Product1/2
  Sum4/1 -> Divide/1
  psi_q_LUT/1 -> Sum5/2  "psi_q_LUT"
  Sum5/1 -> Divide1/1
  psi_d_LUT/1 -> Sum4/2  "psi_d_LUT"
  psi_d_set/1 -> Sum4/1  "psi_d_set"
  psi_q_set/1 -> Sum5/1  "psi_q_set"
  Divide/1 -> Scope/1, Ldd/1, Switch/1  "Ldd"
  Divide1/1 -> Scope/2, Lqq/1, Switch1/1  "Lqq"
  e_id/1 -> Switch2/1, Abs/1  "error_id"
  Constant4/1 -> Switch2/3
  Abs/1 -> Switch2/2
  Switch2/1 -> Divide/2
  e_iq/1 -> Switch3/1, Abs1/1  "error_id"
  Switch3/1 -> Divide1/2
  Abs1/1 -> Switch3/2
  Constant5/1 -> Switch3/3

== system gm_uz_pmsm_model_6LUT_pd_vnl/uz_pmsm_model/Abs ==
  In1 : Inport
  Abs : Abs  SampleTime=1e-08  OutDataTypeStr=single  SaturateOnIntegerOverflow=off
  Out1 : Outport
  wires:
  Abs/1 -> Out1/1
  In1/1 -> Abs/1

== system gm_uz_pmsm_model_6LUT_pd_vnl/uz_pmsm_model/Divide ==
  In1 : Inport
  In2 : Inport  Port=2
  Divide : Product  Inputs=**  OutDataTypeStr=single  SampleTime=1e-08
  Divide_pd1 : Delay  DelayLength=6
  Out1 : Outport
  wires:
  Divide_pd1/1 -> Out1/1
  Divide/1 -> Divide_pd1/1
  In2/1 -> Divide/2
  In1/1 -> Divide/1

== system gm_uz_pmsm_model_6LUT_pd_vnl/uz_pmsm_model/Divide1 ==
  In1 : Inport
  In2 : Inport  Port=2
  Divide1 : Product  Inputs=*/  OutDataTypeStr=single  SampleTime=1e-08
  Divide1_pd1 : Delay  DelayLength=17
  Out1 : Outport
  wires:
  Divide1_pd1/1 -> Out1/1
  Divide1/1 -> Divide1_pd1/1
  In2/1 -> Divide1/2
  In1/1 -> Divide1/1

== system gm_uz_pmsm_model_6LUT_pd_vnl/uz_pmsm_model/Divide_recip ==
  In1 : Inport
  Divide_recip : Math  Operator=reciprocal  SampleTime=1e-08
  Divide_recip_pd1 : Delay  DelayLength=16
  Out1 : Outport
  wires:
  Divide_recip_pd1/1 -> Out1/1
  Divide_recip/1 -> Divide_recip_pd1/1
  In1/1 -> Divide_recip/1

== system gm_uz_pmsm_model_6LUT_pd_vnl/uz_pmsm_model/Factor ==
  In1 : Inport
  In2 : Inport  Port=2
  Factor : Product  Inputs=**  OutDataTypeStr=single  SampleTime=1e-08
  Factor_pd1 : Delay  DelayLength=6
  Out1 : Outport
  wires:
  Factor_pd1/1 -> Out1/1
  Factor/1 -> Factor_pd1/1
  In2/1 -> Factor/2
  In1/1 -> Factor/1

== system gm_uz_pmsm_model_6LUT_pd_vnl/uz_pmsm_model/Gain ==
  In1 : Inport
  In2 : Inport  Port=2
  Gain : Product  Inputs=**  OutDataTypeStr=single  SampleTime=1e-08
  Gain_pd1 : Delay  DelayLength=6
  Out1 : Outport
  wires:
  Gain_pd1/1 -> Out1/1
  Gain/1 -> Gain_pd1/1
  In2/1 -> Gain/2
  In1/1 -> Gain/1

== system gm_uz_pmsm_model_6LUT_pd_vnl/uz_pmsm_model/Gain7 ==
  In1 : Inport
  In2 : Inport  Port=2
  Gain7 : Product  Inputs=**  OutDataTypeStr=single  SampleTime=1e-08
  Gain7_pd1 : Delay  DelayLength=6
  Out1 : Outport
  wires:
  Gain7_pd1/1 -> Out1/1
  Gain7/1 -> Gain7_pd1/1
  In2/1 -> Gain7/2
  In1/1 -> Gain7/1

== system gm_uz_pmsm_model_6LUT_pd_vnl/uz_pmsm_model/Gain71 ==
  In1 : Inport
  In2 : Inport  Port=2
  Gain71 : Product  Inputs=**  OutDataTypeStr=single  SampleTime=1e-08
  Gain71_pd1 : Delay  DelayLength=6
  Out1 : Outport
  wires:
  Gain71_pd1/1 -> Out1/1
  Gain71/1 -> Gain71_pd1/1
  In2/1 -> Gain71/2
  In1/1 -> Gain71/1

== system gm_uz_pmsm_model_6LUT_pd_vnl/uz_pmsm_model/Gain_unaryminus ==
  In1 : Inport
  Gain_unaryminus : UnaryMinus  SampleTime=1e-08
  Out1 : Outport
  wires:
  Gain_unaryminus/1 -> Out1/1
  In1/1 -> Gain_unaryminus/1

== system gm_uz_pmsm_model_6LUT_pd_vnl/uz_pmsm_model/Gain_unaryminus1 ==
  In1 : Inport
  Gain_unaryminus1 : UnaryMinus  SampleTime=1e-08
  Out1 : Outport
  wires:
  Gain_unaryminus1/1 -> Out1/1
  In1/1 -> Gain_unaryminus1/1

== system gm_uz_pmsm_model_6LUT_pd_vnl/uz_pmsm_model/Log ==
  In1 : Inport
  Log : Math  Operator=log  SampleTime=1e-08
  Log_pd1 : Delay  DelayLength=20
  Out1 : Outport
  wires:
  Log_pd1/1 -> Out1/1
  Log/1 -> Log_pd1/1
  In1/1 -> Log/1

== system gm_uz_pmsm_model_6LUT_pd_vnl/uz_pmsm_model/Log1 ==
  In1 : Inport
  Log1 : Math  Operator=log  SampleTime=1e-08
  Log1_pd1 : Delay  DelayLength=20
  Out1 : Outport
  wires:
  Log1_pd1/1 -> Out1/1
  Log1/1 -> Log1_pd1/1
  In1/1 -> Log1/1

== system gm_uz_pmsm_model_6LUT_pd_vnl/uz_pmsm_model/Log11 ==
  In1 : Inport
  Log11 : Math  Operator=log  SampleTime=1e-08
  Log11_pd1 : Delay  DelayLength=20
  Out1 : Outport
  wires:
  Log11_pd1/1 -> Out1/1
  Log11/1 -> Log11_pd1/1
  In1/1 -> Log11/1

== system gm_uz_pmsm_model_6LUT_pd_vnl/uz_pmsm_model/Log2 ==
  In1 : Inport
  Log2 : Math  Operator=log  SampleTime=1e-08
  Log2_pd1 : Delay  DelayLength=20
  Out1 : Outport
  wires:
  Log2_pd1/1 -> Out1/1
  Log2/1 -> Log2_pd1/1
  In1/1 -> Log2/1

== system gm_uz_pmsm_model_6LUT_pd_vnl/uz_pmsm_model/Product ==
  In1 : Inport
  In2 : Inport  Port=2
  Product : Product  Inputs=**  OutDataTypeStr=single  SampleTime=1e-08
  Product_pd1 : Delay  DelayLength=6
  Out1 : Outport
  wires:
  Product_pd1/1 -> Out1/1
  Product/1 -> Product_pd1/1
  In2/1 -> Product/2
  In1/1 -> Product/1

== system gm_uz_pmsm_model_6LUT_pd_vnl/uz_pmsm_model/Product1 ==
  In1 : Inport
  In2 : Inport  Port=2
  Product1 : Product  Inputs=**  OutDataTypeStr=single  SampleTime=1e-08
  Product1_pd1 : Delay  DelayLength=6
  Out1 : Outport
  wires:
  Product1_pd1/1 -> Out1/1
  Product1/1 -> Product1_pd1/1
  In2/1 -> Product1/2
  In1/1 -> Product1/1

== system gm_uz_pmsm_model_6LUT_pd_vnl/uz_pmsm_model/Product10 ==
  In1 : Inport
  In2 : Inport  Port=2
  Product10 : Product  Inputs=**  OutDataTypeStr=single  SampleTime=1e-08
  Product10_pd1 : Delay  DelayLength=6
  Out1 : Outport
  wires:
  Product10_pd1/1 -> Out1/1
  Product10/1 -> Product10_pd1/1
  In2/1 -> Product10/2
  In1/1 -> Product10/1

== system gm_uz_pmsm_model_6LUT_pd_vnl/uz_pmsm_model/Product101 ==
  In1 : Inport
  In2 : Inport  Port=2
  Product101 : Product  Inputs=**  OutDataTypeStr=single  SampleTime=1e-08
  Product101_pd1 : Delay  DelayLength=6
  Out1 : Outport
  wires:
  Product101_pd1/1 -> Out1/1
  Product101/1 -> Product101_pd1/1
  In2/1 -> Product101/2
  In1/1 -> Product101/1

== system gm_uz_pmsm_model_6LUT_pd_vnl/uz_pmsm_model/Product102 ==
  In1 : Inport
  In2 : Inport  Port=2
  Product102 : Product  Inputs=**  OutDataTypeStr=single  SampleTime=1e-08
  Product102_pd1 : Delay  DelayLength=6
  Out1 : Outport
  wires:
  Product102_pd1/1 -> Out1/1
  Product102/1 -> Product102_pd1/1
  In2/1 -> Product102/2
  In1/1 -> Product102/1

== system gm_uz_pmsm_model_6LUT_pd_vnl/uz_pmsm_model/Product103 ==
  In1 : Inport
  In2 : Inport  Port=2
  Product103 : Product  Inputs=**  OutDataTypeStr=single  SampleTime=1e-08
  Product103_pd1 : Delay  DelayLength=6
  Out1 : Outport
  wires:
  Product103_pd1/1 -> Out1/1
  Product103/1 -> Product103_pd1/1
  In2/1 -> Product103/2
  In1/1 -> Product103/1

== system gm_uz_pmsm_model_6LUT_pd_vnl/uz_pmsm_model/Product104 ==
  In1 : Inport
  In2 : Inport  Port=2
  Product104 : Product  Inputs=**  OutDataTypeStr=single  SampleTime=1e-08
  Product104_pd1 : Delay  DelayLength=6
  Out1 : Outport
  wires:
  Product104_pd1/1 -> Out1/1
  Product104/1 -> Product104_pd1/1
  In2/1 -> Product104/2
  In1/1 -> Product104/1

== system gm_uz_pmsm_model_6LUT_pd_vnl/uz_pmsm_model/Product11 ==
  In1 : Inport
  In2 : Inport  Port=2
  Product11 : Product  Inputs=**  OutDataTypeStr=single  SampleTime=1e-08
  Product11_pd1 : Delay  DelayLength=6
  Out1 : Outport
  wires:
  Product11_pd1/1 -> Out1/1
  Product11/1 -> Product11_pd1/1
  In2/1 -> Product11/2
  In1/1 -> Product11/1
